simulink model "dz_2"  (R2023a)
settings: Solver=ode23s  StartTime=0.0  StopTime=300  MinStep=1e-4  RelTol=1e-3
libraries: simulink x2
settings Model: Creator=diontep  LastModifiedBy=diontep

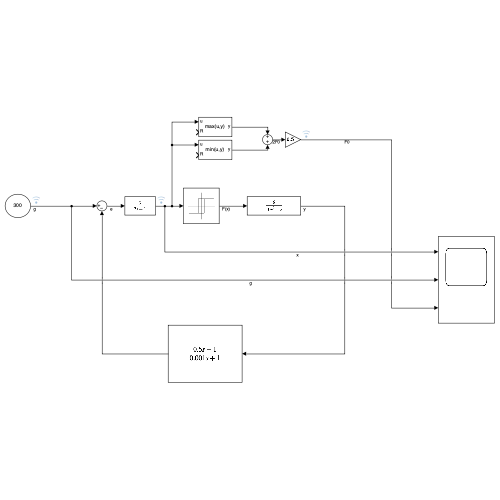
[thumbnail: Simulink's stored preview of the top-level diagram]
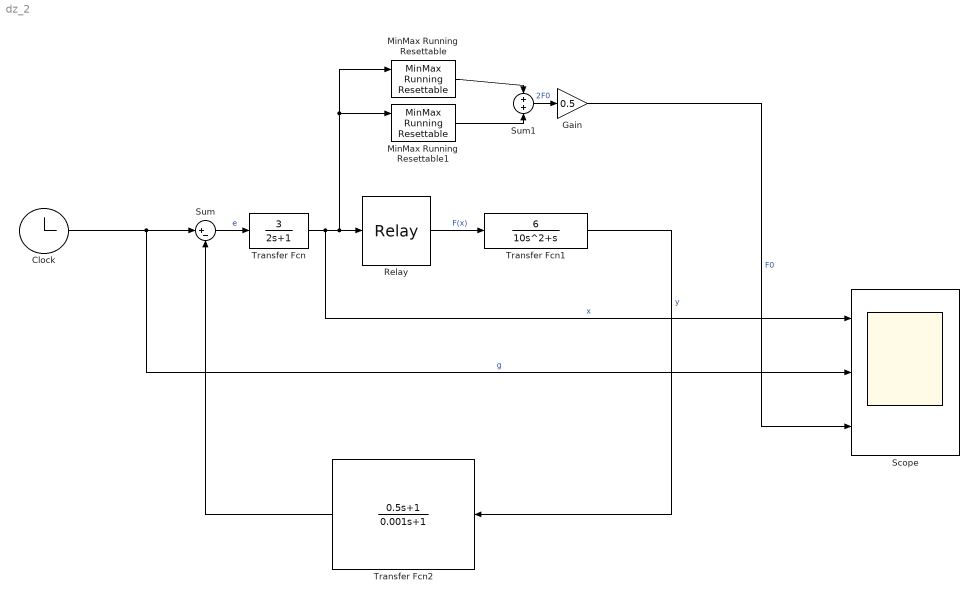
== system dz_2 ==
  Clock : Clock
  Gain : Gain  Gain=0.5
  MinMax Running Resettable : simulink/Math Operations/MinMax Running Resettable  Function=max  vinit=0.0
  MinMax Running Resettable1 : simulink/Math Operations/MinMax Running Resettable  Function=min  vinit=0.0
  Relay : Relay  OnSwitchValue=0  OffSwitchValue=0  OnOutputValue=pi/2  OffOutputValue=-pi/2
  Scope : Scope  NumInputPorts=3
  Sum : Sum  Inputs=|+-
  Sum1 : Sum
  Transfer Fcn : TransferFcn  Numerator=[3]  Denominator=[2 1]
  Transfer Fcn1 : TransferFcn  Numerator=[6]  Denominator=[10 1 0]
  Transfer Fcn2 : TransferFcn  Numerator=[0.5 1]  Denominator=[0.001 1]
  wires:
  Clock/1 -> Scope/2, Sum/1  "g"
  Sum/1 -> Transfer Fcn/1  "e"
  Transfer Fcn/1 -> MinMax Running Resettable1/1, MinMax Running Resettable/1, Relay/1, Scope/1  "x"
  Relay/1 -> Transfer Fcn1/1  "F(x)"
  Transfer Fcn1/1 -> Transfer Fcn2/1  "y"
  Transfer Fcn2/1 -> Sum/2
  MinMax Running Resettable/1 -> Sum1/1
  MinMax Running Resettable1/1 -> Sum1/2
  Sum1/1 -> Gain/1  "2F0"
  Gain/1 -> Scope/3  "F0"
